simulink model "NMPC_PH"  (R2021a)
settings: Solver=VariableStepAuto  StartTime=0.0  StopTime=100  RelTol=1e-3
values from neighbouring files (symbols this model uses):
  Ts = 0.5    [NonlinearMPC_PH.m]    (also in TITO_ph_StateFcnDT.m)
  u0 = 0.1    [NonlinearMPC_PH.m]
undefined symbols (not defined in the file or in its folder): sigbuilder_block
libraries: sharedTrackingLibrary x1, mpclib x1, simulink x1
settings Model: Creator=CHEMENG  LastModifiedBy=USER

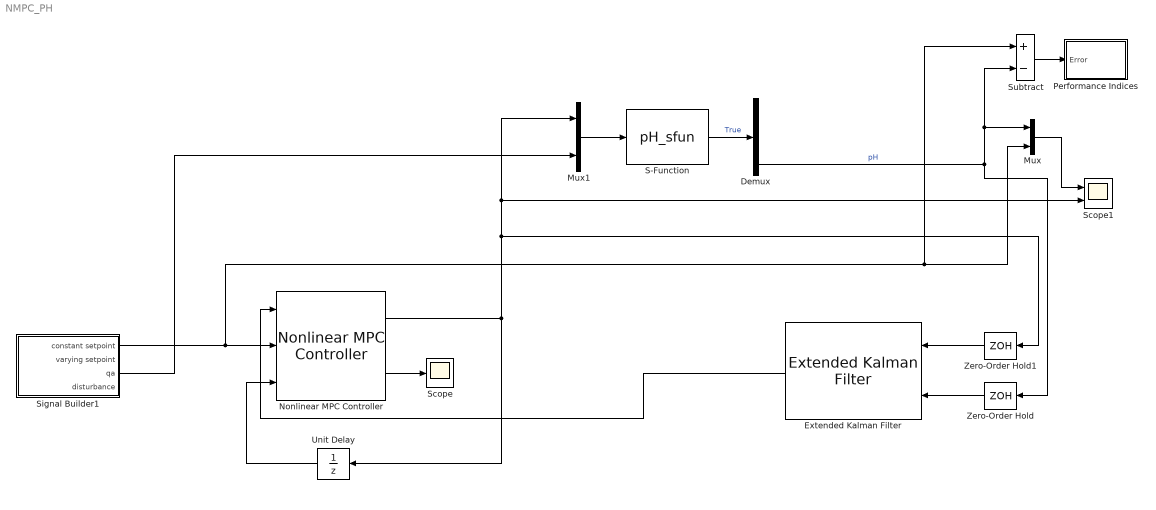
== system NMPC_PH ==
  Demux : Demux
  Extended Kalman Filter : sharedTrackingLibrary/Extended Kalman Filter  StateTransitionFcn=TITO_ph_StateFcnDT  HasStateTransitionJacobianFcn=off  HasAdditiveProcessNoise=Additive  ProcessNoise=[1e-3]  HasTimeVaryingProcessNoise=off  HasStateTransitionFcnExtraArgument=1  InitialState=x0  InitialStateCovariance=[1e-3]  MeasurementFcn1=TITO_ph_MeasFcn  HasMeasurementJacobianFcn1=off  HasMeasurementEnablePort1=off  HasAdditiveMeasurementNoise1=Additive  MeasurementNoise1=[1e-3]  HasTimeVaryingMeasurementNoise1=off  HasMeasurementFcnExtraArgument1=0  MeasurementFcn2=myMeasurementFcn  HasMeasurementJacobianFcn2=off  HasMeasurementEnablePort2=off  HasAdditiveMeasurementNoise2=Additive  MeasurementNoise2=1  HasTimeVaryingMeasurementNoise2=off  HasMeasurementFcnExtraArgument2=0  MeasurementFcn3=myMeasurementFcn  HasMeasurementJacobianFcn3=off  HasMeasurementEnablePort3=off  HasAdditiveMeasurementNoise3=Additive  MeasurementNoise3=1  HasTimeVaryingMeasurementNoise3=off  HasMeasurementFcnExtraArgument3=0  MeasurementFcn4=myMeasurementFcn  HasMeasurementJacobianFcn4=off  HasMeasurementEnablePort4=off  HasAdditiveMeasurementNoise4=Additive  MeasurementNoise4=1  HasTimeVaryingMeasurementNoise4=off  HasMeasurementFcnExtraArgument4=0  MeasurementFcn5=myMeasurementFcn  HasMeasurementJacobianFcn5=off  HasMeasurementEnablePort5=off  HasAdditiveMeasurementNoise5=Additive  MeasurementNoise5=1  HasTimeVaryingMeasurementNoise5=off  HasMeasurementFcnExtraArgument5=0  EnableMultirate=off  StateTransitionFcnSampleTime=1  MeasurementFcn1SampleTime=1  MeasurementFcn2SampleTime=1  MeasurementFcn3SampleTime=1  MeasurementFcn4SampleTime=1  MeasurementFcn5SampleTime=1  UseCurrentEstimator=on  OutputStateCovariance=off  DataType=double  SampleTime=Ts  NumberOfMeasurements=1
      settings: SourceProductBaseCode=CT,DR,TF,ID,LP,NV,AR,RO,RR,UV,VE
  Mux : Mux  Inputs=2
  Mux1 : Mux  Inputs=2
  Nonlinear MPC Controller : mpclib/Nonlinear MPC Controller  SCDEnableBlockLinearizationSpecification=on  nlmpcobj=nlobj  UseObjectTs=on  UseMEX=off  md_enabled=off  mvtarget_enabled=off  param_enabled=off  cost_enabled=off  mvseq_enabled=off  stateseq_enabled=off  ovseq_enabled=off  slack_enabled=off  status_enabled=on  ov_min=off  ov_max=off  mv_min=off  mv_max=off  mvrate_min=off  mvrate_max=off  state_min=off  state_max=off  ov_weight=off  mv_weight=off  mvrate_weight=off  ecr_weight=off  nlp_initialize=off
  Performance Indices : Subsystem
  S-Function : S-Function  FunctionName=pH_sfun  SFunctionDeploymentMode=off  EnableBusSupport=off
  Scope : Scope
  Scope1 : Scope  NumInputPorts=2
  Signal Builder1 : Subsystem  Tag=STV Subsys  LoadFcn=sigbuilder_block('load');  StartFcn=sigbuilder_block('start');  StopFcn=sigbuilder_block('stop');  ClipboardFcn=sigbuilder_block('clipboard');  mask(Sigbuilder block){tuvar=[0:10]}
      mask help: Simulink:masks:SigbuilderBlock_MD
      mask init:
      | if ~strcmp(get_param(bdroot(gcbh),'SimulationStatus'),'stopped') tuvar = sigbuilder_block('maskInit'); end
      settings: CopyFcn=sigbuilder_block('copy');  DeleteFcn=sigbuilder_block('delete');  ModelCloseFcn=sigbuilder_block('modelClose');  PreSaveFcn=sigbuilder_block('preSave');  PauseFcn=sigbuilder_block('pause');  ContinueFcn=sigbuilder_block('continue');  NameChangeFcn=sigbuilder_block('namechange');  OpenFcn=sigbuilder_block('open',[379.5 6 575 469 ]);  CloseFcn=sigbuilder_block('close');
      mask Display: plot(0, 0, 100, 100,[2, 2, 32, 32, 2], [68, 8, 8, 68, 68],[32, 2], [38, 38], [32, 19, 2],[53, 60, 44], [32, 17, 17, 2],[16, 16, 31, 31]);txt = getActiveGroup(gcbh);text(2, 100, txt,'verticalAlignment', 'top');
  Subtract : Sum  Inputs=+-
  Unit Delay : UnitDelay  InitialCondition=u0  SampleTime=-1  HasFrameUpgradeWarning=on
  Zero-Order Hold : ZeroOrderHold  SampleTime=Ts
  Zero-Order Hold1 : ZeroOrderHold  SampleTime=Ts
  wires:
  Nonlinear MPC Controller/1 -> Scope1/2, Mux1/1, Zero-Order Hold1/1, Unit Delay/1
  Unit Delay/1 -> Nonlinear MPC Controller/3
  Zero-Order Hold/1 -> Extended Kalman Filter/2
  Zero-Order Hold1/1 -> Extended Kalman Filter/1
  Extended Kalman Filter/1 -> Nonlinear MPC Controller/1
  Nonlinear MPC Controller/2 -> Scope/1
  Mux1/1 -> S-Function/1
  Signal Builder1/3(qa) -> Mux1/2
  S-Function/1 -> Demux/1  "True"
  Mux/1 -> Scope1/1
  Subtract/1 -> Performance Indices/1(Error)
  Demux/4 -> Subtract/2, Mux/1, Zero-Order Hold/1  "pH"
  Signal Builder1/1(constant setpoint) -> Subtract/1, Mux/2, Nonlinear MPC Controller/2

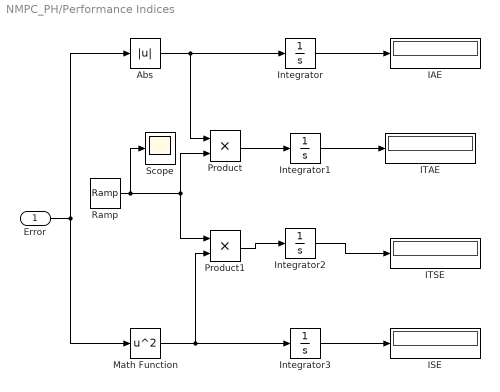
== system NMPC_PH/Performance Indices ==
  Error : Inport
  Abs : Abs
  IAE : Display
  ISE : Display
  ITAE : Display
  ITSE : Display
  Integrator{,1..3} (4 alike) : Integrator
  Math Function : Math  Operator=square  SignedPower=on  SaturateOnIntegerOverflow=on
  Product : Product  RndMeth=Zero
  Product1 : Product  RndMeth=Zero
  Ramp : simulink/Sources/Ramp  slope=1  start=0  InitialOutput=0
  Scope : Scope
  wires:
  Error/1 -> Math Function/1, Abs/1
  Abs/1 -> Integrator/1, Product/1
  Integrator/1 -> IAE/1
  Ramp/1 -> Product/2, Product1/1, Scope/1
  Math Function/1 -> Integrator3/1, Product1/2
  Product1/1 -> Integrator2/1
  Product/1 -> Integrator1/1
  Integrator3/1 -> ISE/1
  Integrator2/1 -> ITSE/1
  Integrator1/1 -> ITAE/1

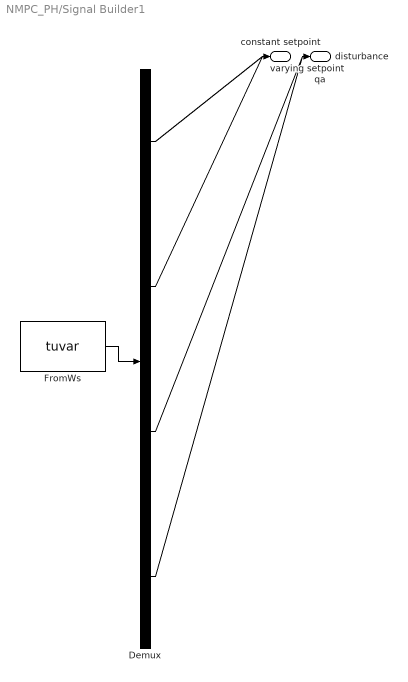
== system NMPC_PH/Signal Builder1 ==
  Demux : Demux  Tag=STV Demux
      settings: DisplayOption=none
  FromWs : FromWorkspace  Tag=STV FromWs  VariableName=tuvar
      SigBuilderData=|
      | common.afterFinalStr = 'Extrapolate'
      | common.sampleTime = 0
      | dataSet(1).timeRange = [0 100]
      | dataSet(1).name = 'Servo'
      | dataSet(2).timeRange = [0 100]
      | dataSet(2).name = 'Regulatory'
      | sbobj.Groups(1).Name = 'Servo'
      | sbobj.Groups(1).Signals(1).Name = 'constant setpoint'
      | sbobj.Groups(1).Signals(1).XData = [0 100]
      | sbobj.Groups(1).Signals(1).YData = [7 7]
      | sbobj.Groups(1).Signals(2).Name = 'varying setpoint'
      | sbobj.Groups(1).Signals(2).XData = [0 10 10 20 20 30 30 40 40 50 50 60 60 70 70 100]
      | sbobj.Groups(1).Signals(2).YData = [3.14776 3.14776 5 5 6 6 7 7 8 8 9 9 10 10 5 5]
      | sbobj.Groups(1).Signals(3).Name = 'qa'
      | sbobj.Groups(1).Signals(3).XData = [0 100]
      | sbobj.Groups(1).Signals(3).YData = [1 1]
      | sbobj.Groups(1).Signals(4).Name = 'disturbance'
      | sbobj.Groups(1).Signals(4).XData = [0 10 10 20 20 30 30 40 40 50 50 60 60 70 70 80 80 90 90 100]
      | sbobj.Groups(1).Signals(4).YData = [1 1 1.5 1.5 1 1 0.5 0.5 1.5 1.5 1 1 0.5 0.5 1.5 1.5 1 1 0.5 0.5]
      | sbobj.Groups(1).TimeRange = [0 100]
      | sbobj.Groups(2).Name = 'Regulatory'
      | sbobj.Groups(2).Signals(1).Name = 'constant setpoint'
      | sbobj.Groups(2).Signals(1).XData = [0 10 10 20 20 30 30 40 40 50 50 100]
      | sbobj.Groups(2).Signals(1).YData = [1 1 1.5 1.5 1 1 0.5 0.5 1.5 1.5 1 1]
      | sbobj.Groups(2).Signals(2).Name = 'varying setpoint'
      | sbobj.Groups(2).Signals(2).XData = [0 100]
      | sbobj.Groups(2).Signals(2).YData = [7.01 7.01]
      | sbobj.Groups(2).Signals(3).Name = 'qa'
      | sbobj.Groups(2).Signals(3).XData = [0 100]
      | sbobj.Groups(2).Signals(3).YData = [0 0]
      | sbobj.Groups(2).Signals(4).Name = 'disturbance'
      | sbobj.Groups(2).Signals(4).XData = [0 100]
      | sbobj.Groups(2).Signals(4).YData = [0 0]
      | sbobj.Groups(2).TimeRange = [0 100]
  constant setpoint : Outport  Tag=STV Outport  VectorParamsAs1DForOutWhenUnconnected=off
  varying setpoint : Outport  Tag=STV Outport  Port=2  VectorParamsAs1DForOutWhenUnconnected=off
  qa : Outport  Tag=STV Outport  Port=3
  disturbance : Outport  Tag=STV Outport  Port=4
  wires:
  FromWs/1 -> Demux/1
  Demux/1 -> constant setpoint/1
  Demux/2 -> varying setpoint/1
  Demux/3 -> qa/1
  Demux/4 -> disturbance/1
